simulink library "REXduino_library"  (Simulink 3.00)
libraries: logiclib x194, mathlib x116, analoglib x15, genlib x12, speclib x4
(part 2 of 2)

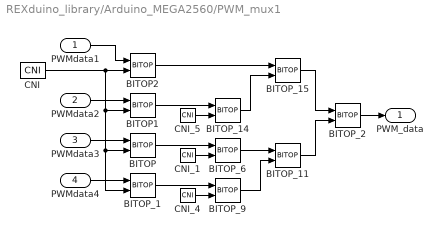
== system REXduino_library/Arduino_MEGA2560/PWM_mux1 ==
  PWMdata1 : Inport  Port=1  PortWidth=-1  SampleTime=-1  DataType=auto
      settings: SignalType=auto
  PWMdata2 : Inport  Port=2  PortWidth=-1  SampleTime=-1  DataType=auto
      settings: SignalType=auto
  PWMdata3 : Inport  Port=3  PortWidth=-1  SampleTime=-1  DataType=auto
      settings: SignalType=auto
  PWMdata4 : Inport  Port=4  PortWidth=-1  SampleTime=-1  DataType=auto
      settings: SignalType=auto
  BITOP : logiclib/BITOP  iop=3: Bit AND
  BITOP1 : logiclib/BITOP  iop=3: Bit AND
  BITOP2 : logiclib/BITOP  iop=3: Bit AND
  BITOP_1 : logiclib/BITOP  iop=3: Bit AND
  BITOP_11 : logiclib/BITOP  iop=2: Bit OR
  BITOP_14 : logiclib/BITOP  iop=5: Shift Left
  BITOP_15 : logiclib/BITOP  iop=2: Bit OR
  BITOP_2 : logiclib/BITOP  iop=2: Bit OR
  BITOP_6 : logiclib/BITOP  iop=5: Shift Left
  BITOP_9 : logiclib/BITOP  iop=5: Shift Left
  CNI : mathlib/CNI  icn=255
  CNI_1 : mathlib/CNI  icn=16
  CNI_4 : mathlib/CNI  icn=24
  CNI_5 : mathlib/CNI  icn=8
  PWM_data : Outport  Port=1
  wires:
  BITOP/1 -> BITOP_6/1
  BITOP1/1 -> BITOP_14/1
  BITOP2/1 -> BITOP_15/1
  BITOP_1/1 -> BITOP_9/1
  BITOP_11/1 -> BITOP_2/2
  BITOP_14/1 -> BITOP_15/2
  BITOP_15/1 -> BITOP_2/1
  BITOP_2/1 -> PWM_data/1
  BITOP_6/1 -> BITOP_11/1
  BITOP_9/1 -> BITOP_11/2
  CNI/1 -> BITOP2/2, BITOP/2, BITOP_1/2, BITOP1/2
  CNI_1/1 -> BITOP_6/2
  CNI_4/1 -> BITOP_9/2
  CNI_5/1 -> BITOP_14/2
  PWMdata1/1 -> BITOP2/1
  PWMdata2/1 -> BITOP1/1
  PWMdata3/1 -> BITOP/1
  PWMdata4/1 -> BITOP_1/1

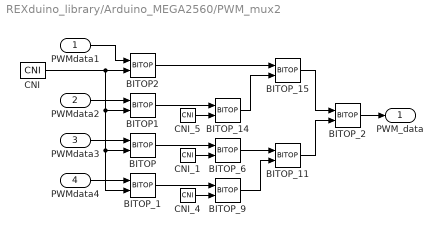
== system REXduino_library/Arduino_MEGA2560/PWM_mux2 ==
  PWMdata1 : Inport  Port=1  PortWidth=-1  SampleTime=-1  DataType=auto
      settings: SignalType=auto
  PWMdata2 : Inport  Port=2  PortWidth=-1  SampleTime=-1  DataType=auto
      settings: SignalType=auto
  PWMdata3 : Inport  Port=3  PortWidth=-1  SampleTime=-1  DataType=auto
      settings: SignalType=auto
  PWMdata4 : Inport  Port=4  PortWidth=-1  SampleTime=-1  DataType=auto
      settings: SignalType=auto
  BITOP : logiclib/BITOP  iop=3: Bit AND
  BITOP1 : logiclib/BITOP  iop=3: Bit AND
  BITOP2 : logiclib/BITOP  iop=3: Bit AND
  BITOP_1 : logiclib/BITOP  iop=3: Bit AND
  BITOP_11 : logiclib/BITOP  iop=2: Bit OR
  BITOP_14 : logiclib/BITOP  iop=5: Shift Left
  BITOP_15 : logiclib/BITOP  iop=2: Bit OR
  BITOP_2 : logiclib/BITOP  iop=2: Bit OR
  BITOP_6 : logiclib/BITOP  iop=5: Shift Left
  BITOP_9 : logiclib/BITOP  iop=5: Shift Left
  CNI : mathlib/CNI  icn=255
  CNI_1 : mathlib/CNI  icn=16
  CNI_4 : mathlib/CNI  icn=24
  CNI_5 : mathlib/CNI  icn=8
  PWM_data : Outport  Port=1
  wires:
  BITOP/1 -> BITOP_6/1
  BITOP1/1 -> BITOP_14/1
  BITOP2/1 -> BITOP_15/1
  BITOP_1/1 -> BITOP_9/1
  BITOP_11/1 -> BITOP_2/2
  BITOP_14/1 -> BITOP_15/2
  BITOP_15/1 -> BITOP_2/1
  BITOP_2/1 -> PWM_data/1
  BITOP_6/1 -> BITOP_11/1
  BITOP_9/1 -> BITOP_11/2
  CNI/1 -> BITOP1/2, BITOP/2, BITOP_1/2, BITOP2/2
  CNI_1/1 -> BITOP_6/2
  CNI_4/1 -> BITOP_9/2
  CNI_5/1 -> BITOP_14/2
  PWMdata1/1 -> BITOP2/1
  PWMdata2/1 -> BITOP1/1
  PWMdata3/1 -> BITOP/1
  PWMdata4/1 -> BITOP_1/1

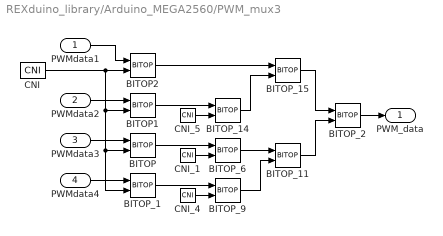
== system REXduino_library/Arduino_MEGA2560/PWM_mux3 ==
  PWMdata1 : Inport  Port=1  PortWidth=-1  SampleTime=-1  DataType=auto
      settings: SignalType=auto
  PWMdata2 : Inport  Port=2  PortWidth=-1  SampleTime=-1  DataType=auto
      settings: SignalType=auto
  PWMdata3 : Inport  Port=3  PortWidth=-1  SampleTime=-1  DataType=auto
      settings: SignalType=auto
  PWMdata4 : Inport  Port=4  PortWidth=-1  SampleTime=-1  DataType=auto
      settings: SignalType=auto
  BITOP : logiclib/BITOP  iop=3: Bit AND
  BITOP1 : logiclib/BITOP  iop=3: Bit AND
  BITOP2 : logiclib/BITOP  iop=3: Bit AND
  BITOP_1 : logiclib/BITOP  iop=3: Bit AND
  BITOP_11 : logiclib/BITOP  iop=2: Bit OR
  BITOP_14 : logiclib/BITOP  iop=5: Shift Left
  BITOP_15 : logiclib/BITOP  iop=2: Bit OR
  BITOP_2 : logiclib/BITOP  iop=2: Bit OR
  BITOP_6 : logiclib/BITOP  iop=5: Shift Left
  BITOP_9 : logiclib/BITOP  iop=5: Shift Left
  CNI : mathlib/CNI  icn=255
  CNI_1 : mathlib/CNI  icn=16
  CNI_4 : mathlib/CNI  icn=24
  CNI_5 : mathlib/CNI  icn=8
  PWM_data : Outport  Port=1
  wires:
  BITOP/1 -> BITOP_6/1
  BITOP1/1 -> BITOP_14/1
  BITOP2/1 -> BITOP_15/1
  BITOP_1/1 -> BITOP_9/1
  BITOP_11/1 -> BITOP_2/2
  BITOP_14/1 -> BITOP_15/2
  BITOP_15/1 -> BITOP_2/1
  BITOP_2/1 -> PWM_data/1
  BITOP_6/1 -> BITOP_11/1
  BITOP_9/1 -> BITOP_11/2
  CNI/1 -> BITOP1/2, BITOP/2, BITOP_1/2, BITOP2/2
  CNI_1/1 -> BITOP_6/2
  CNI_4/1 -> BITOP_9/2
  CNI_5/1 -> BITOP_14/2
  PWMdata1/1 -> BITOP2/1
  PWMdata2/1 -> BITOP1/1
  PWMdata3/1 -> BITOP/1
  PWMdata4/1 -> BITOP_1/1

== system REXduino_library/Arduino_MEGA2560/Simulation_Detector ==
  CNI3 : mathlib/CNI  icn=1
  Y : Outport  Port=1
  wires:
  CNI3/1 -> Y/1

== system REXduino_library/Arduino_MEGA2560hex/CNT_mux ==
  CNT2R : Inport  Port=1  PortWidth=-1  SampleTime=-1  DataType=auto
      settings: SignalType=auto
  CNT2E : Inport  Port=2  PortWidth=-1  SampleTime=-1  DataType=auto
      settings: SignalType=auto
  CNT3R : Inport  Port=3  PortWidth=-1  SampleTime=-1  DataType=auto
      settings: SignalType=auto
  CNT3E : Inport  Port=4  PortWidth=-1  SampleTime=-1  DataType=auto
      settings: SignalType=auto
  OCTBM : logiclib/BMOCT  shift=0
  cntCmd : Outport  Port=1
  wires:
  CNT2E/1 -> OCTBM/2
  CNT2R/1 -> OCTBM/1
  CNT3E/1 -> OCTBM/4
  CNT3R/1 -> OCTBM/3
  OCTBM/1 -> cntCmd/1

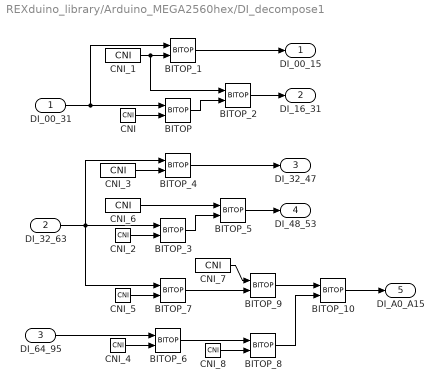
== system REXduino_library/Arduino_MEGA2560hex/DI_decompose1 ==
  DI_00_31 : Inport  Port=1  PortWidth=-1  SampleTime=-1  DataType=auto
      settings: SignalType=auto
  DI_32_63 : Inport  Port=2  PortWidth=-1  SampleTime=-1  DataType=auto
      settings: SignalType=auto
  DI_64_95 : Inport  Port=3  PortWidth=-1  SampleTime=-1  DataType=auto
      settings: SignalType=auto
  BITOP : logiclib/BITOP  iop=6: Shift Right
  BITOP_{1..2,4..6,9} (6 alike) : logiclib/BITOP  iop=3: Bit AND
  BITOP_10 : logiclib/BITOP  iop=2: Bit OR
  BITOP_3 : logiclib/BITOP  iop=6: Shift Right
  BITOP_7 : logiclib/BITOP  iop=6: Shift Right
  BITOP_8 : logiclib/BITOP  iop=5: Shift Left
  CNI : mathlib/CNI  icn=16
  CNI_1 : mathlib/CNI  icn=65535
  CNI_2 : mathlib/CNI  icn=16
  CNI_3 : mathlib/CNI  icn=65535
  CNI_4 : mathlib/CNI  icn=63
  CNI_5 : mathlib/CNI  icn=22
  CNI_6 : mathlib/CNI  icn=63
  CNI_7 : mathlib/CNI  icn=1023
  CNI_8 : mathlib/CNI  icn=10
  DI_00_15 : Outport  Port=1
  DI_16_31 : Outport  Port=2
  DI_32_47 : Outport  Port=3
  DI_48_53 : Outport  Port=4
  DI_A0_A15 : Outport  Port=5
  wires:
  BITOP/1 -> BITOP_2/2
  BITOP_1/1 -> DI_00_15/1
  BITOP_10/1 -> DI_A0_A15/1
  BITOP_2/1 -> DI_16_31/1
  BITOP_3/1 -> BITOP_5/2
  BITOP_4/1 -> DI_32_47/1
  BITOP_5/1 -> DI_48_53/1
  BITOP_6/1 -> BITOP_8/1
  BITOP_7/1 -> BITOP_9/2
  BITOP_8/1 -> BITOP_10/2
  BITOP_9/1 -> BITOP_10/1
  CNI/1 -> BITOP/2
  CNI_1/1 -> BITOP_1/2, BITOP_2/1
  CNI_2/1 -> BITOP_3/2
  CNI_3/1 -> BITOP_4/2
  CNI_4/1 -> BITOP_6/2
  CNI_5/1 -> BITOP_7/2
  CNI_6/1 -> BITOP_5/1
  CNI_7/1 -> BITOP_9/1
  CNI_8/1 -> BITOP_8/2
  DI_00_31/1 -> BITOP/1, BITOP_1/1
  DI_32_63/1 -> BITOP_3/1, BITOP_4/1, BITOP_7/1
  DI_64_95/1 -> BITOP_6/1

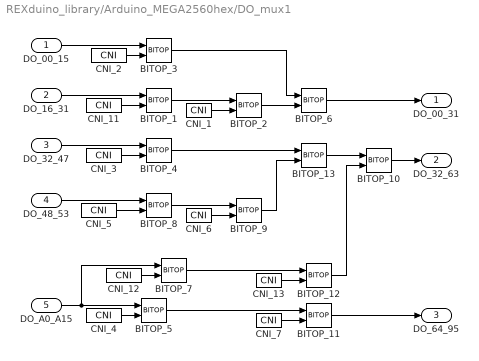
== system REXduino_library/Arduino_MEGA2560hex/DO_mux1 ==
  DO_00_15 : Inport  Port=1  PortWidth=-1  SampleTime=-1  DataType=auto
      settings: SignalType=auto
  DO_16_31 : Inport  Port=2  PortWidth=-1  SampleTime=-1  DataType=auto
      settings: SignalType=auto
  DO_32_47 : Inport  Port=3  PortWidth=-1  SampleTime=-1  DataType=auto
      settings: SignalType=auto
  DO_48_53 : Inport  Port=4  PortWidth=-1  SampleTime=-1  DataType=auto
      settings: SignalType=auto
  DO_A0_A15 : Inport  Port=5  PortWidth=-1  SampleTime=-1  DataType=auto
      settings: SignalType=auto
  BITOP_{1,3..5,7..8} (6 alike) : logiclib/BITOP  iop=3: Bit AND
  BITOP_10 : logiclib/BITOP  iop=2: Bit OR
  BITOP_11 : logiclib/BITOP  iop=6: Shift Right
  BITOP_12 : logiclib/BITOP  iop=5: Shift Left
  BITOP_13 : logiclib/BITOP  iop=2: Bit OR
  BITOP_2 : logiclib/BITOP  iop=5: Shift Left
  BITOP_6 : logiclib/BITOP  iop=2: Bit OR
  BITOP_9 : logiclib/BITOP  iop=5: Shift Left
  CNI_1 : mathlib/CNI  icn=16
  CNI_11 : mathlib/CNI  icn=65535
  CNI_12 : mathlib/CNI  icn=1023
  CNI_13 : mathlib/CNI  icn=22
  CNI_2 : mathlib/CNI  icn=65535
  CNI_3 : mathlib/CNI  icn=65535
  CNI_4 : mathlib/CNI  icn=64512
  CNI_5 : mathlib/CNI  icn=63
  CNI_6 : mathlib/CNI  icn=16
  CNI_7 : mathlib/CNI  icn=10
  DO_00_31 : Outport  Port=1
  DO_32_63 : Outport  Port=2
  DO_64_95 : Outport  Port=3
  wires:
  BITOP_1/1 -> BITOP_2/1
  BITOP_10/1 -> DO_32_63/1
  BITOP_11/1 -> DO_64_95/1
  BITOP_12/1 -> BITOP_10/2
  BITOP_13/1 -> BITOP_10/1
  BITOP_2/1 -> BITOP_6/2
  BITOP_3/1 -> BITOP_6/1
  BITOP_4/1 -> BITOP_13/1
  BITOP_5/1 -> BITOP_11/1
  BITOP_6/1 -> DO_00_31/1
  BITOP_7/1 -> BITOP_12/1
  BITOP_8/1 -> BITOP_9/1
  BITOP_9/1 -> BITOP_13/2
  CNI_1/1 -> BITOP_2/2
  CNI_11/1 -> BITOP_1/2
  CNI_12/1 -> BITOP_7/2
  CNI_13/1 -> BITOP_12/2
  CNI_2/1 -> BITOP_3/2
  CNI_3/1 -> BITOP_4/2
  CNI_4/1 -> BITOP_5/2
  CNI_5/1 -> BITOP_8/2
  CNI_6/1 -> BITOP_9/2
  CNI_7/1 -> BITOP_11/2
  DO_00_15/1 -> BITOP_3/1
  DO_16_31/1 -> BITOP_1/1
  DO_32_47/1 -> BITOP_4/1
  DO_48_53/1 -> BITOP_8/1
  DO_A0_A15/1 -> BITOP_5/1, BITOP_7/1

== system REXduino_library/Arduino_MEGA2560hex/ERR_demux ==
  data : Inport  Port=1  PortWidth=-1  SampleTime=-1  DataType=auto
      settings: SignalType=auto
  BITOP_1 : logiclib/BITOP  iop=6: Shift Right
  BITOP_{2,4,6,10} (4 alike) : logiclib/BITOP  iop=3: Bit AND
  BITOP_5 : logiclib/BITOP  iop=6: Shift Right
  BITOP_7 : logiclib/BITOP  iop=6: Shift Right
  CNI : mathlib/CNI  icn=255
  CNI_1 : mathlib/CNI  icn=8
  CNI_2 : mathlib/CNI  icn=63
  CNI_3 : mathlib/CNI  icn=6
  CNI_4 : mathlib/CNI  icn=1023
  err_code : Outport  Port=1
  err_subcode : Outport  Port=2
  status : Outport  Port=3
  AIdata : Outport  Port=4
  wires:
  BITOP_1/1 -> BITOP_2/1, BITOP_5/1
  BITOP_10/1 -> err_subcode/1
  BITOP_2/1 -> err_code/1
  BITOP_4/1 -> AIdata/1
  BITOP_5/1 -> BITOP_6/1, BITOP_7/1
  BITOP_6/1 -> status/1
  BITOP_7/1 -> BITOP_4/1
  CNI/1 -> BITOP_10/2, BITOP_2/2
  CNI_1/1 -> BITOP_1/2, BITOP_5/2
  CNI_2/1 -> BITOP_6/2
  CNI_3/1 -> BITOP_7/2
  CNI_4/1 -> BITOP_4/2
  data/1 -> BITOP_1/1, BITOP_10/1

== system REXduino_library/Arduino_MEGA2560hex/Simulation_Detector ==
  CNI3 : mathlib/CNI  icn=1
  Y : Outport  Port=1
  wires:
  CNI3/1 -> Y/1

== system REXduino_library/Arduino_UNO/AI_demux1 ==
  AI_data : Inport  Port=1  PortWidth=-1  SampleTime=-1  DataType=auto
      settings: SignalType=auto
  BITOP_1 : logiclib/BITOP  iop=6: Shift Right
  BITOP_10 : logiclib/BITOP  iop=3: Bit AND
  BITOP_2 : logiclib/BITOP  iop=3: Bit AND
  BITOP_3 : logiclib/BITOP  iop=6: Shift Right
  BITOP_4 : logiclib/BITOP  iop=3: Bit AND
  CNI : mathlib/CNI  icn=1023
  CNI_1 : mathlib/CNI  icn=10
  AIdata1 : Outport  Port=1
  AIdata2 : Outport  Port=2
  AIdata3 : Outport  Port=3
  wires:
  AI_data/1 -> BITOP_1/1, BITOP_10/1
  BITOP_1/1 -> BITOP_2/1, BITOP_3/1
  BITOP_10/1 -> AIdata1/1
  BITOP_2/1 -> AIdata2/1
  BITOP_3/1 -> BITOP_4/1
  BITOP_4/1 -> AIdata3/1
  CNI/1 -> BITOP_10/2, BITOP_2/2, BITOP_4/2
  CNI_1/1 -> BITOP_1/2, BITOP_3/2

== system REXduino_library/Arduino_UNO/AI_demux2 ==
  AI_data : Inport  Port=1  PortWidth=-1  SampleTime=-1  DataType=auto
      settings: SignalType=auto
  BITOP_1 : logiclib/BITOP  iop=6: Shift Right
  BITOP_10 : logiclib/BITOP  iop=3: Bit AND
  BITOP_2 : logiclib/BITOP  iop=3: Bit AND
  BITOP_3 : logiclib/BITOP  iop=6: Shift Right
  BITOP_4 : logiclib/BITOP  iop=3: Bit AND
  CNI : mathlib/CNI  icn=1023
  CNI_1 : mathlib/CNI  icn=10
  AIdata1 : Outport  Port=1
  AIdata2 : Outport  Port=2
  AIdata3 : Outport  Port=3
  wires:
  AI_data/1 -> BITOP_1/1, BITOP_10/1
  BITOP_1/1 -> BITOP_2/1, BITOP_3/1
  BITOP_10/1 -> AIdata1/1
  BITOP_2/1 -> AIdata2/1
  BITOP_3/1 -> BITOP_4/1
  BITOP_4/1 -> AIdata3/1
  CNI/1 -> BITOP_10/2, BITOP_2/2, BITOP_4/2
  CNI_1/1 -> BITOP_1/2, BITOP_3/2

== system REXduino_library/Arduino_UNO/CNT_mux ==
  CNT2R : Inport  Port=1  PortWidth=-1  SampleTime=-1  DataType=auto
      settings: SignalType=auto
  CNT2E : Inport  Port=2  PortWidth=-1  SampleTime=-1  DataType=auto
      settings: SignalType=auto
  CNT3R : Inport  Port=3  PortWidth=-1  SampleTime=-1  DataType=auto
      settings: SignalType=auto
  CNT3E : Inport  Port=4  PortWidth=-1  SampleTime=-1  DataType=auto
      settings: SignalType=auto
  OCTBM : logiclib/BMOCT  shift=0
  cntCmd : Outport  Port=1
  wires:
  CNT2E/1 -> OCTBM/2
  CNT2R/1 -> OCTBM/1
  CNT3E/1 -> OCTBM/4
  CNT3R/1 -> OCTBM/3
  OCTBM/1 -> cntCmd/1

== system REXduino_library/Arduino_UNO/ERR_demux ==
  data : Inport  Port=1  PortWidth=-1  SampleTime=-1  DataType=auto
      settings: SignalType=auto
  BITOP_1 : logiclib/BITOP  iop=6: Shift Right
  BITOP_{2,4,6,10} (4 alike) : logiclib/BITOP  iop=3: Bit AND
  BITOP_5 : logiclib/BITOP  iop=6: Shift Right
  BITOP_7 : logiclib/BITOP  iop=6: Shift Right
  CNI : mathlib/CNI  icn=255
  CNI_1 : mathlib/CNI  icn=8
  CNI_2 : mathlib/CNI  icn=63
  CNI_3 : mathlib/CNI  icn=6
  CNI_4 : mathlib/CNI  icn=1023
  err_code : Outport  Port=1
  err_subcode : Outport  Port=2
  status : Outport  Port=3
  AIdata : Outport  Port=4
  wires:
  BITOP_1/1 -> BITOP_2/1, BITOP_5/1
  BITOP_10/1 -> err_subcode/1
  BITOP_2/1 -> err_code/1
  BITOP_4/1 -> AIdata/1
  BITOP_5/1 -> BITOP_6/1, BITOP_7/1
  BITOP_6/1 -> status/1
  BITOP_7/1 -> BITOP_4/1
  CNI/1 -> BITOP_10/2, BITOP_2/2
  CNI_1/1 -> BITOP_1/2, BITOP_5/2
  CNI_2/1 -> BITOP_6/2
  CNI_3/1 -> BITOP_7/2
  CNI_4/1 -> BITOP_4/2
  data/1 -> BITOP_1/1, BITOP_10/1

== system REXduino_library/Arduino_UNO/Simulation_Detector ==
  CNI3 : mathlib/CNI  icn=1
  Y : Outport  Port=1
  wires:
  CNI3/1 -> Y/1

== system REXduino_library/Arduino_UNOhex/AI_demux1 ==
  AI_data : Inport  Port=1  PortWidth=-1  SampleTime=-1  DataType=auto
      settings: SignalType=auto
  BITOP_1 : logiclib/BITOP  iop=6: Shift Right
  BITOP_10 : logiclib/BITOP  iop=3: Bit AND
  BITOP_2 : logiclib/BITOP  iop=3: Bit AND
  BITOP_3 : logiclib/BITOP  iop=6: Shift Right
  BITOP_4 : logiclib/BITOP  iop=3: Bit AND
  CNI : mathlib/CNI  icn=1023
  CNI_1 : mathlib/CNI  icn=10
  AIdata1 : Outport  Port=1
  AIdata2 : Outport  Port=2
  AIdata3 : Outport  Port=3
  wires:
  AI_data/1 -> BITOP_1/1, BITOP_10/1
  BITOP_1/1 -> BITOP_2/1, BITOP_3/1
  BITOP_10/1 -> AIdata1/1
  BITOP_2/1 -> AIdata2/1
  BITOP_3/1 -> BITOP_4/1
  BITOP_4/1 -> AIdata3/1
  CNI/1 -> BITOP_10/2, BITOP_2/2, BITOP_4/2
  CNI_1/1 -> BITOP_1/2, BITOP_3/2

== system REXduino_library/Arduino_UNOhex/AI_demux2 ==
  AI_data : Inport  Port=1  PortWidth=-1  SampleTime=-1  DataType=auto
      settings: SignalType=auto
  BITOP_1 : logiclib/BITOP  iop=6: Shift Right
  BITOP_10 : logiclib/BITOP  iop=3: Bit AND
  BITOP_2 : logiclib/BITOP  iop=3: Bit AND
  BITOP_3 : logiclib/BITOP  iop=6: Shift Right
  BITOP_4 : logiclib/BITOP  iop=3: Bit AND
  CNI : mathlib/CNI  icn=1023
  CNI_1 : mathlib/CNI  icn=10
  AIdata1 : Outport  Port=1
  AIdata2 : Outport  Port=2
  AIdata3 : Outport  Port=3
  wires:
  AI_data/1 -> BITOP_1/1, BITOP_10/1
  BITOP_1/1 -> BITOP_2/1, BITOP_3/1
  BITOP_10/1 -> AIdata1/1
  BITOP_2/1 -> AIdata2/1
  BITOP_3/1 -> BITOP_4/1
  BITOP_4/1 -> AIdata3/1
  CNI/1 -> BITOP_10/2, BITOP_2/2, BITOP_4/2
  CNI_1/1 -> BITOP_1/2, BITOP_3/2

== system REXduino_library/Arduino_UNOhex/CNT_mux ==
  CNT2R : Inport  Port=1  PortWidth=-1  SampleTime=-1  DataType=auto
      settings: SignalType=auto
  CNT2E : Inport  Port=2  PortWidth=-1  SampleTime=-1  DataType=auto
      settings: SignalType=auto
  CNT3R : Inport  Port=3  PortWidth=-1  SampleTime=-1  DataType=auto
      settings: SignalType=auto
  CNT3E : Inport  Port=4  PortWidth=-1  SampleTime=-1  DataType=auto
      settings: SignalType=auto
  OCTBM : logiclib/BMOCT  shift=0
  cntCmd : Outport  Port=1
  wires:
  CNT2E/1 -> OCTBM/2
  CNT2R/1 -> OCTBM/1
  CNT3E/1 -> OCTBM/4
  CNT3R/1 -> OCTBM/3
  OCTBM/1 -> cntCmd/1

== system REXduino_library/Arduino_UNOhex/ERR_demux ==
  data : Inport  Port=1  PortWidth=-1  SampleTime=-1  DataType=auto
      settings: SignalType=auto
  BITOP_1 : logiclib/BITOP  iop=6: Shift Right
  BITOP_{2,4,6,10} (4 alike) : logiclib/BITOP  iop=3: Bit AND
  BITOP_5 : logiclib/BITOP  iop=6: Shift Right
  BITOP_7 : logiclib/BITOP  iop=6: Shift Right
  CNI : mathlib/CNI  icn=255
  CNI_1 : mathlib/CNI  icn=8
  CNI_2 : mathlib/CNI  icn=63
  CNI_3 : mathlib/CNI  icn=6
  CNI_4 : mathlib/CNI  icn=1023
  err_code : Outport  Port=1
  err_subcode : Outport  Port=2
  status : Outport  Port=3
  AIdata : Outport  Port=4
  wires:
  BITOP_1/1 -> BITOP_2/1, BITOP_5/1
  BITOP_10/1 -> err_subcode/1
  BITOP_2/1 -> err_code/1
  BITOP_4/1 -> AIdata/1
  BITOP_5/1 -> BITOP_6/1, BITOP_7/1
  BITOP_6/1 -> status/1
  BITOP_7/1 -> BITOP_4/1
  CNI/1 -> BITOP_10/2, BITOP_2/2
  CNI_1/1 -> BITOP_1/2, BITOP_5/2
  CNI_2/1 -> BITOP_6/2
  CNI_3/1 -> BITOP_7/2
  CNI_4/1 -> BITOP_4/2
  data/1 -> BITOP_1/1, BITOP_10/1

== system REXduino_library/Arduino_UNOhex/Simulation_Detector ==
  CNI3 : mathlib/CNI  icn=1
  Y : Outport  Port=1
  wires:
  CNI3/1 -> Y/1
